simulink model "foot"  (R2014b)
settings: Solver=ode45  StartTime=0.0  StopTime=1  RelTol=1e-3
undefined symbols (not defined in the file or in its folder): MX28_inertia, MX28_Te, X, Y, Z
libraries: sm_lib x10, nesl_utility x7
settings Model: Creator=florent  LastModifiedBy=florent
settings DebuggingCC: IntegerOverflowMsg=none  ParameterDowncastMsg=warning  ParameterPrecisionLossMsg=none  ParameterTunabilityLossMsg=none  StateNameClashWarn=warning  IntegerSaturationMsg=none

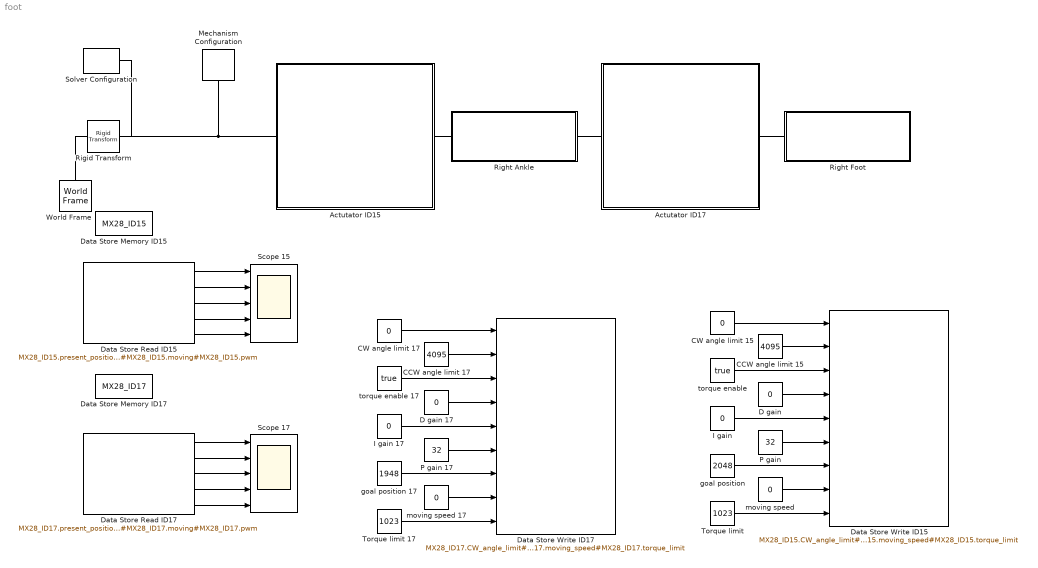
== system foot ==
  Actutator ID15 : Subsystem
  Actutator ID17 : Subsystem
  CCW angle limit 15 : Constant  Value=4095  OutDataTypeStr=int16
  CCW angle limit 17 : Constant  Value=4095  OutDataTypeStr=int16
  CW angle limit 15 : Constant  Value=0  OutDataTypeStr=int16
  CW angle limit 17 : Constant  Value=0  OutDataTypeStr=int16
  D gain : Constant  Value=0  OutDataTypeStr=uint8
  D gain 17 : Constant  Value=0  OutDataTypeStr=uint8
  Data Store Memory ID15 : DataStoreMemory  DataStoreName=MX28_ID15  WriteAfterWriteMsg=error  InitialValue=MX28_default  VectorParams1D=off  OutDataTypeStr=Bus: MX28_bus
  Data Store Memory ID17 : DataStoreMemory  DataStoreName=MX28_ID17  WriteAfterWriteMsg=error  InitialValue=MX28_default  VectorParams1D=off  OutDataTypeStr=Bus: MX28_bus
  Data Store Read ID15 : DataStoreRead  DataStoreName=MX28_ID15  SampleTime=0.001  DataStoreElements=MX28_ID15.present_position#MX28_ID15.present_speed#MX28_ID15.present_load#MX28_ID15.moving#MX28_ID15.pwm
  Data Store Read ID17 : DataStoreRead  DataStoreName=MX28_ID17  SampleTime=0.001  DataStoreElements=MX28_ID17.present_position#MX28_ID17.present_speed#MX28_ID17.present_load#MX28_ID17.moving#MX28_ID17.pwm
  Data Store Write ID15 : DataStoreWrite  DataStoreName=MX28_ID15  DataStoreElements=MX28_ID15.CW_angle_limit#MX28_ID15.CCW_angle_limit#MX28_ID15.torque_enable#MX28_ID15.D_gain#MX28_ID15.I_gain#MX28_ID15.P_gain#MX28_ID15.goal_position#MX28_ID15.moving_speed#MX28_ID15.torque_limit
  Data Store Write ID17 : DataStoreWrite  DataStoreName=MX28_ID17  DataStoreElements=MX28_ID17.CW_angle_limit#MX28_ID17.CCW_angle_limit#MX28_ID17.torque_enable#MX28_ID17.D_gain#MX28_ID17.I_gain#MX28_ID17.P_gain#MX28_ID17.goal_position#MX28_ID17.moving_speed#MX28_ID17.torque_limit
  I gain : Constant  Value=0  OutDataTypeStr=uint8
  I gain 17 : Constant  Value=0  OutDataTypeStr=uint8
  Mechanism Configuration : sm_lib/Utilities/Mechanism Configuration  UniformGravity=Constant  GravityVector=[0 -9.80665 0]  GravityUnits=m/s^2  LinearizationDelta=0.001  BlockFunction=simmechanics.library.utilities.mechanism_configuration
  P gain : Constant  Value=32  OutDataTypeStr=uint8
  P gain 17 : Constant  Value=32  OutDataTypeStr=uint8
  Right Ankle : Subsystem
      mask init:
      | [ModelDir,~,~] = fileparts(which(gcs));
      | 
      | Block = [gcb '/Solid'];
      | STLFileName = [ModelDir filesep 'STL' filesep 'Right_Ankle.STL'];
      | if ~strcmp(get_param(Block,'ExtGeomFileName'),STLFileName)
      |     set_param(Block,'ExtGeomFileName',STLFileName);
      | end
  Right Foot : Subsystem
      mask init:
      | [ModelDir,~,~] = fileparts(which(gcs));
      | 
      | Block = [gcb '/Solid'];
      | STLFileName = [ModelDir filesep 'STL' filesep 'Right_Foot.STL'];
      | if ~strcmp(get_param(Block,'ExtGeomFileName'),STLFileName)
      |     set_param(Block,'ExtGeomFileName',STLFileName);
      | end
  Rigid Transform : sm_lib/Frames and Transforms/Rigid Transform  TranslationMethod=Cartesian  TranslationLengthUnit=m  TranslationStandardAxis=+Z  TranslationStandardOffset=0  TranslationCartesianOffset=[0 -0.001 0]  TranslationROffset=0  TranslationROffsetUnits=m  TranslationZOffset=0  TranslationZOffsetUnits=m  TranslationThetaOffset=0  TranslationThetaOffsetUnits=deg  RotationMethod=AlignedAxes  RotationAngleUnits=deg  RotationStandardAxis=+Z  RotationAngle=0  RotationArbitraryAxis=[0 0 1]  FollAlignAxisA=+Z  BaseAlignAxisA=+X  FollAlignAxisB=+Y  BaseAlignAxisB=+Z  RotationMatrix=[1 0 0; 0 1 0; 0 0 1]  BlockFunction=simmechanics.library.frames_transforms.rigid_transform
  Scope 15 : Scope  NumInputPorts=5
      settings: YMin=-5~0~-5~-5~-5  YMax=5~650~5~5~5
  Scope 17 : Scope  NumInputPorts=5
      settings: YMin=-5~0~-5~-5~-5  YMax=5~650~5~5~5
  Solver Configuration : nesl_utility/Solver Configuration  PhysicalDomain=network_engine_domain  SubClassName=solver  LeftPortType=input  RightPortType=generic  Accelerate=off  Tones=[]  Harmonics=[]  SimulateNoise=off  Profile=off  UseLocalSampling=off  EnableSwitchedLinearOptims=on  FrequencyDomain=off  UseCCode=off  RelTol=0.001  AbsTol=1e-06  MinStep=1e-09  ToWorkspace=off  DoDC=off  ResidualTolerance=1e-09  UseLocalSolver=off  LocalSolverChoice=NE_BACKWARD_EULER_ADVANCER  LocalSolverSampleTime=0.001  DoFixedCost=off  MaxNonlinIter=3  MaxModeIter=2  LinearAlgebra=Sparse  DelaysMemoryBudget=1024  AutomaticFiltering=on  FilteringTimeConstant=0.001
  Torque limit : Constant  Value=1023  OutDataTypeStr=int16
  Torque limit 17 : Constant  Value=1023  OutDataTypeStr=int16
  World Frame : sm_lib/Frames and Transforms/World Frame  BlockFunction=simmechanics.library.frames_transforms.world_frame
  goal position : Constant  Value=2048  OutDataTypeStr=int16
  goal position 17 : Constant  Value=1948  OutDataTypeStr=int16
  moving speed : Constant  Value=0  OutDataTypeStr=int16
  moving speed 17 : Constant  Value=0  OutDataTypeStr=int16
  torque enable : Constant  Value=true  OutDataTypeStr=boolean
  torque enable 17 : Constant  Value=true  OutDataTypeStr=boolean
  wires:
  Data Store Read ID15/1 -> Scope 15/1
  Data Store Read ID15/2 -> Scope 15/2
  Data Store Read ID15/3 -> Scope 15/3
  Data Store Read ID15/4 -> Scope 15/4
  Data Store Read ID15/5 -> Scope 15/5
  Data Store Read ID17/1 -> Scope 17/1
  Data Store Read ID17/2 -> Scope 17/2
  Data Store Read ID17/3 -> Scope 17/3
  Data Store Read ID17/4 -> Scope 17/4
  Data Store Read ID17/5 -> Scope 17/5
  Torque limit 17/1 -> Data Store Write ID17/9
  moving speed 17/1 -> Data Store Write ID17/8
  goal position 17/1 -> Data Store Write ID17/7
  P gain 17/1 -> Data Store Write ID17/6
  I gain 17/1 -> Data Store Write ID17/5
  D gain 17/1 -> Data Store Write ID17/4
  torque enable 17/1 -> Data Store Write ID17/3
  CW angle limit 17/1 -> Data Store Write ID17/1
  CCW angle limit 17/1 -> Data Store Write ID17/2
  Torque limit/1 -> Data Store Write ID15/9
  moving speed/1 -> Data Store Write ID15/8
  goal position/1 -> Data Store Write ID15/7
  P gain/1 -> Data Store Write ID15/6
  I gain/1 -> Data Store Write ID15/5
  D gain/1 -> Data Store Write ID15/4
  torque enable/1 -> Data Store Write ID15/3
  CCW angle limit 15/1 -> Data Store Write ID15/2
  CW angle limit 15/1 -> Data Store Write ID15/1
  connections:
  Mechanism Configuration/RConn1 -- Rigid Transform/RConn1 -- Solver Configuration/RConn1 -- Actutator ID15/LConn1
  Actutator ID15/RConn1 -- Right Ankle/LConn1
  Actutator ID17/LConn1 -- Right Ankle/RConn1
  Actutator ID17/RConn1 -- Right Foot/LConn1
  Rigid Transform/LConn1 -- World Frame/RConn1

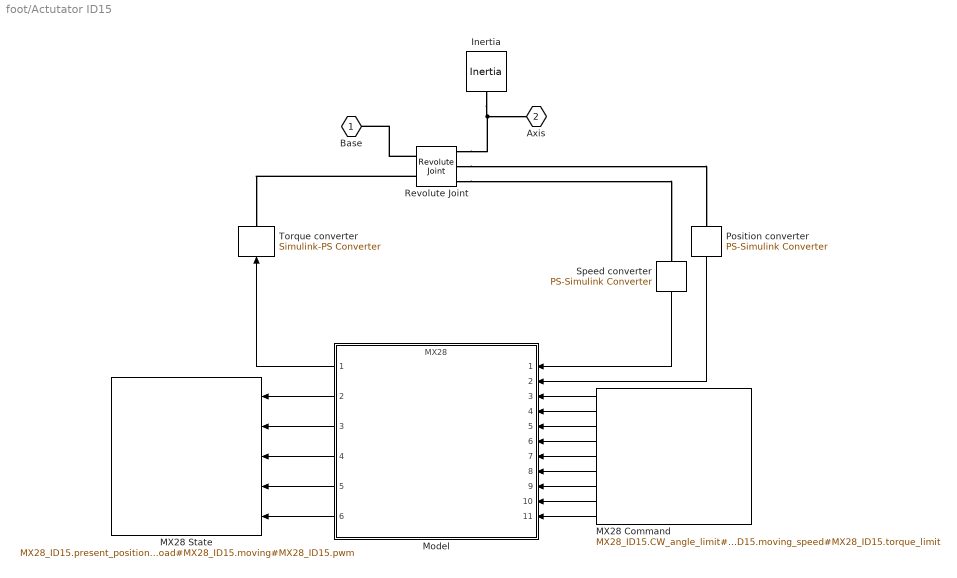
== system foot/Actutator ID15 ==
  Inertia : sm_lib/Body Elements/Inertia  InertiaType=Custom  Mass=1  MassUnits=g  CenterOfMass=[0 0 0]  CenterOfMassUnits=m  MomentsOfInertia=[0 0 MX28_inertia]  MomentsOfInertiaUnits=kg*m^2  ProductsOfInertia=[0 0 0]  ProductsOfInertiaUnits=kg*m^2  BlockFunction=simmechanics.library.body_elements.inertia
  MX28 Command : DataStoreRead  DataStoreName=MX28_ID15  SampleTime=MX28_Te  DataStoreElements=MX28_ID15.CW_angle_limit#MX28_ID15.CCW_angle_limit#MX28_ID15.torque_enable#MX28_ID15.D_gain#MX28_ID15.I_gain#MX28_ID15.P_gain#MX28_ID15.goal_position#MX28_ID15.moving_speed#MX28_ID15.torque_limit
  MX28 State : DataStoreWrite  DataStoreName=MX28_ID15  DataStoreElements=MX28_ID15.present_position#MX28_ID15.present_speed#MX28_ID15.present_load#MX28_ID15.moving#MX28_ID15.pwm
  Model : ModelReference  ModelNameDialog=MX28.slx  SimulationMode=Normal  ModelReferenceVersion=1.66  CopyOfModelName=MX28.slx  DefaultDataLogging=on
  Position converter : nesl_utility/PS-Simulink Converter  PhysicalDomain=network_engine_domain  SubClassName=ps_output  LeftPortType=input  RightPortType=output  PseudoPeriodic=off  Frequencies=[]  Unit=rad  AffineConversion=off
  Revolute Joint : sm_lib/Joints/Revolute Joint  SenseConstraintForce=off  SenseConstraintForceX=off  SenseConstraintForceY=off  SenseConstraintForceZ=off  SenseConstraintTorque=off  SenseConstraintTorqueX=off  SenseConstraintTorqueY=off  SenseConstraintTorqueZ=off  SenseTotalForce=off  SenseTotalForceX=off  SenseTotalForceY=off  SenseTotalForceZ=off  SenseTotalTorque=off  SenseTotalTorqueX=off  SenseTotalTorqueY=off  SenseTotalTorqueZ=off  CompositeWrenchDir=FollowerOnBase  CompositeWrenchFrame=BaseFrame  EquilibriumPosition=0  EquilibriumPositionUnits=deg  SpringStiffness=0  SpringStiffnessUnits=N*m/deg  DampingCoefficient=MX28_lub_friction  DampingCoefficientUnits=N*m/(rad/s)  TorqueActuationMode=InputTorque  MotionActuationMode=ComputedMotion  SensePosition=on  SenseVelocity=on  SenseAcceleration=off  SenseTorqueForce=off  PositionTargetValue=MX28_init_position  PositionTargetValueUnits=rad  PositionTargetSpecify=on  PositionTargetPriority=High  VelocityTargetValue=MX28_init_speed  VelocityTargetValueUnits=rad/s  VelocityTargetSpecify=on  VelocityTargetPriority=High  BlockFunction=simmechanics.library.joints.revolute_joint
  Speed converter : nesl_utility/PS-Simulink Converter  PhysicalDomain=network_engine_domain  SubClassName=ps_output  LeftPortType=input  RightPortType=output  PseudoPeriodic=off  Frequencies=[]  Unit=rad/s  AffineConversion=off
  Torque converter : nesl_utility/Simulink-PS Converter  PhysicalDomain=network_engine_domain  SubClassName=ps_input  LeftPortType=input  RightPortType=output  PseudoPeriodic=off  Frequencies=[]  NoiseDistribution=none  NoiseParameters=[]  Unit=N*m  AffineConversion=off  InputFiltering=off  SimscapeFilterOrder=1  InputFilterTimeConstant=0.001  UdotUserProvided=1
  Base : PMIOPort  Port=1  Side=Left
  Axis : PMIOPort  Port=2  Side=Right
  wires:
  Model/4 -> MX28 State/3
  Model/2 -> MX28 State/1
  Model/5 -> MX28 State/4
  Model/3 -> MX28 State/2
  Model/1 -> Torque converter/1
  Speed converter/1 -> Model/1
  Position converter/1 -> Model/2
  MX28 Command/3 -> Model/5
  MX28 Command/6 -> Model/8
  MX28 Command/4 -> Model/6
  MX28 Command/5 -> Model/7
  MX28 Command/7 -> Model/9
  MX28 Command/2 -> Model/4
  MX28 Command/1 -> Model/3
  Model/6 -> MX28 State/5
  MX28 Command/8 -> Model/10
  MX28 Command/9 -> Model/11
  connections:
  Inertia/RConn1 -- Axis/RConn1 -- Revolute Joint/RConn1
  Revolute Joint/RConn2 -- Position converter/LConn1
  Revolute Joint/LConn2 -- Torque converter/RConn1
  Revolute Joint/RConn3 -- Speed converter/LConn1
  Revolute Joint/LConn1 -- Base/RConn1

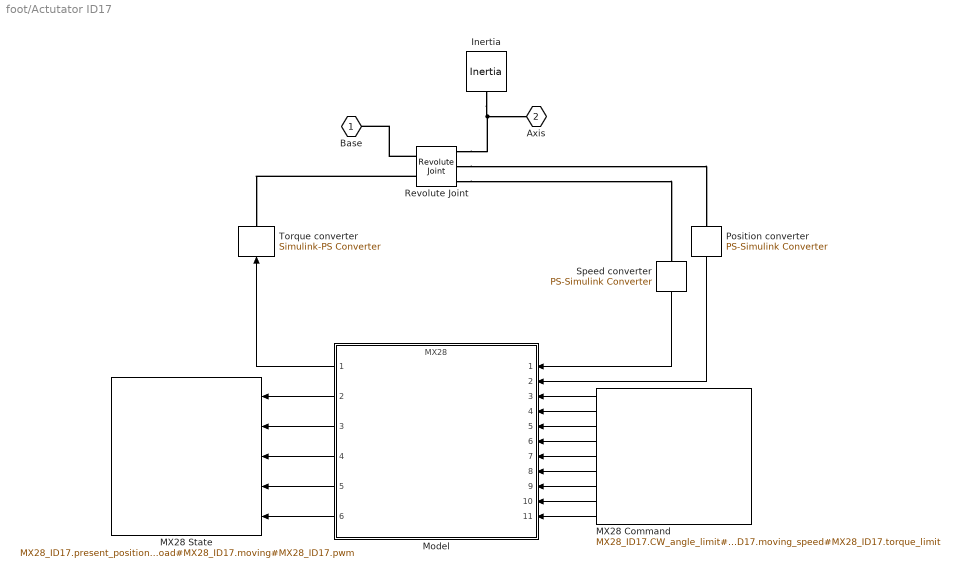
== system foot/Actutator ID17 ==
  Inertia : sm_lib/Body Elements/Inertia  InertiaType=Custom  Mass=1  MassUnits=g  CenterOfMass=[0 0 0]  CenterOfMassUnits=m  MomentsOfInertia=[0 0 MX28_inertia]  MomentsOfInertiaUnits=kg*m^2  ProductsOfInertia=[0 0 0]  ProductsOfInertiaUnits=kg*m^2  BlockFunction=simmechanics.library.body_elements.inertia
  MX28 Command : DataStoreRead  DataStoreName=MX28_ID17  SampleTime=MX28_Te  DataStoreElements=MX28_ID17.CW_angle_limit#MX28_ID17.CCW_angle_limit#MX28_ID17.torque_enable#MX28_ID17.D_gain#MX28_ID17.I_gain#MX28_ID17.P_gain#MX28_ID17.goal_position#MX28_ID17.moving_speed#MX28_ID17.torque_limit
  MX28 State : DataStoreWrite  DataStoreName=MX28_ID17  DataStoreElements=MX28_ID17.present_position#MX28_ID17.present_speed#MX28_ID17.present_load#MX28_ID17.moving#MX28_ID17.pwm
  Model : ModelReference  ModelNameDialog=MX28.slx  SimulationMode=Normal  ModelReferenceVersion=1.66  CopyOfModelName=MX28.slx  DefaultDataLogging=on
  Position converter : nesl_utility/PS-Simulink Converter  PhysicalDomain=network_engine_domain  SubClassName=ps_output  LeftPortType=input  RightPortType=output  PseudoPeriodic=off  Frequencies=[]  Unit=rad  AffineConversion=off
  Revolute Joint : sm_lib/Joints/Revolute Joint  SenseConstraintForce=off  SenseConstraintForceX=off  SenseConstraintForceY=off  SenseConstraintForceZ=off  SenseConstraintTorque=off  SenseConstraintTorqueX=off  SenseConstraintTorqueY=off  SenseConstraintTorqueZ=off  SenseTotalForce=off  SenseTotalForceX=off  SenseTotalForceY=off  SenseTotalForceZ=off  SenseTotalTorque=off  SenseTotalTorqueX=off  SenseTotalTorqueY=off  SenseTotalTorqueZ=off  CompositeWrenchDir=FollowerOnBase  CompositeWrenchFrame=BaseFrame  EquilibriumPosition=0  EquilibriumPositionUnits=deg  SpringStiffness=0  SpringStiffnessUnits=N*m/deg  DampingCoefficient=MX28_lub_friction  DampingCoefficientUnits=N*m/(rad/s)  TorqueActuationMode=InputTorque  MotionActuationMode=ComputedMotion  SensePosition=on  SenseVelocity=on  SenseAcceleration=off  SenseTorqueForce=off  PositionTargetValue=MX28_init_position  PositionTargetValueUnits=rad  PositionTargetSpecify=on  PositionTargetPriority=High  VelocityTargetValue=MX28_init_speed  VelocityTargetValueUnits=rad/s  VelocityTargetSpecify=on  VelocityTargetPriority=High  BlockFunction=simmechanics.library.joints.revolute_joint
  Speed converter : nesl_utility/PS-Simulink Converter  PhysicalDomain=network_engine_domain  SubClassName=ps_output  LeftPortType=input  RightPortType=output  PseudoPeriodic=off  Frequencies=[]  Unit=rad/s  AffineConversion=off
  Torque converter : nesl_utility/Simulink-PS Converter  PhysicalDomain=network_engine_domain  SubClassName=ps_input  LeftPortType=input  RightPortType=output  PseudoPeriodic=off  Frequencies=[]  NoiseDistribution=none  NoiseParameters=[]  Unit=N*m  AffineConversion=off  InputFiltering=off  SimscapeFilterOrder=1  InputFilterTimeConstant=0.001  UdotUserProvided=1
  Base : PMIOPort  Port=1  Side=Left
  Axis : PMIOPort  Port=2  Side=Right
  wires:
  Model/4 -> MX28 State/3
  Model/2 -> MX28 State/1
  Model/5 -> MX28 State/4
  Model/3 -> MX28 State/2
  Model/1 -> Torque converter/1
  Speed converter/1 -> Model/1
  Position converter/1 -> Model/2
  MX28 Command/3 -> Model/5
  MX28 Command/6 -> Model/8
  MX28 Command/4 -> Model/6
  MX28 Command/5 -> Model/7
  MX28 Command/7 -> Model/9
  MX28 Command/2 -> Model/4
  MX28 Command/1 -> Model/3
  Model/6 -> MX28 State/5
  MX28 Command/8 -> Model/10
  MX28 Command/9 -> Model/11
  connections:
  Inertia/RConn1 -- Axis/RConn1 -- Revolute Joint/RConn1
  Revolute Joint/RConn3 -- Speed converter/LConn1
  Revolute Joint/LConn2 -- Torque converter/RConn1
  Revolute Joint/RConn2 -- Position converter/LConn1
  Revolute Joint/LConn1 -- Base/RConn1

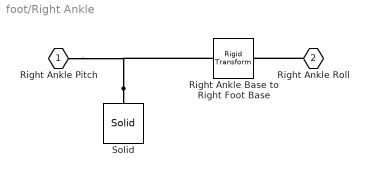
== system foot/Right Ankle ==
  Right Ankle Base to Right Foot Base : sm_lib/Frames and Transforms/Rigid Transform  TranslationMethod=Cartesian  TranslationLengthUnit=mm  TranslationStandardAxis=+Z  TranslationStandardOffset=0  TranslationCartesianOffset=[-19.35 0 -24]  TranslationROffset=0  TranslationROffsetUnits=m  TranslationZOffset=0  TranslationZOffsetUnits=m  TranslationThetaOffset=0  TranslationThetaOffsetUnits=deg  RotationMethod=AlignedAxes  RotationAngleUnits=deg  RotationStandardAxis=+Z  RotationAngle=0  RotationArbitraryAxis=[0 0 1]  FollAlignAxisA=+X  BaseAlignAxisA=+Z  FollAlignAxisB=+Y  BaseAlignAxisB=-Y  RotationMatrix=[1 0 0; 0 1 0; 0 0 1]  BlockFunction=simmechanics.library.frames_transforms.rigid_transform
  Solid : sm_lib/Body Elements/Solid  InertiaType=Custom  Mass=166.79  MassUnits=g  CenterOfMass=[-18.06 -11.21 -24.20]  CenterOfMassUnits=mm  MomentsOfInertia=[6948 12212 11817]  MomentsOfInertiaUnits=g*mm^2  ProductsOfInertia=[-194 117 4006]  ProductsOfInertiaUnits=g*mm^2  DensityBased=on  Density=1000  DensityUnits=kg/(m^3)  GraphicType=FromGeometry  MarkerShape=Sphere  MarkerSize=10  MarkerSizeUnits=m  GraphicVisPropType=SimpleVisualProperties  GraphicDiffuseColor=[0.5 0.5 0.5]  GraphicSpecularColor=[0.5 0.5 0.5 1.0]  GraphicAmbientColor=[0.15 0.15 0.15 1.0]  GraphicEmissiveColor=[0.0 0.0 0.0 1.0]  GraphicShininess=75  GraphicOpacity=1.0  GeometryShape=FromFile  RectangleSize=[1 1]  RectangleSizeUnits=m  BrickDimensions=[1 1 1]  BrickDimensionUnits=m  CylinderRadius=1  CylinderRadiusUnits=m  CylinderLength=1  CylinderLengthUnits=m  SphereRadius=1  SphereRadiusUnits=m  EllipsoidRadii=[1 1 1]  EllipsoidRadiiUnits=m  ExtrusionCrossSection=[1 1; -1 1; -1 -1; 1 -1]  ExtrusionCrossSectionUnits=m  ExtrusionLength=1  ExtrusionLengthUnits=m  PolygonNumSides=3  PolygonOuterRadius=1  PolygonOuterRadiusUnits=m  ExtGeomFileType=STL  ExtGeomFileName=D:\Ker Lann\systemes\darwin\kinematics\STL\Right_Ankle.STL  ExtGeomFileUnits=mm  RevolutionCrossSection=[1 1; 1 -1; 2 -1; 2 1]  RevolutionCrossSectionUnits=m  RevolutionExtent=Full  RevolutionAngle=180  RevolutionAngleUnits=deg  BlockFunction=simmechanics.library.body_elements.solid
  Right Ankle Pitch : PMIOPort  Port=1  Side=Left
  Right Ankle Roll : PMIOPort  Port=2  Side=Right
  connections:
  Solid/RConn1 -- Right Ankle Base to Right Foot Base/LConn1 -- Right Ankle Pitch/RConn1
  Right Ankle Roll/RConn1 -- Right Ankle Base to Right Foot Base/RConn1

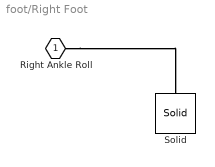
== system foot/Right Foot ==
  Solid : sm_lib/Body Elements/Solid  InertiaType=Custom  Mass=76.78  MassUnits=g  CenterOfMass=[7.76 24.5 17.25]  CenterOfMassUnits=mm  MomentsOfInertia=[69069 85303 36676]  MomentsOfInertiaUnits=g*mm^2  ProductsOfInertia=[4062 778 2754]  ProductsOfInertiaUnits=g*mm^2  DensityBased=on  Density=1000  DensityUnits=kg/(m^3)  GraphicType=FromGeometry  MarkerShape=Sphere  MarkerSize=10  MarkerSizeUnits=m  GraphicVisPropType=SimpleVisualProperties  GraphicDiffuseColor=[0.5 0.5 0.5]  GraphicSpecularColor=[0.5 0.5 0.5 1.0]  GraphicAmbientColor=[0.15 0.15 0.15 1.0]  GraphicEmissiveColor=[0.0 0.0 0.0 1.0]  GraphicShininess=75  GraphicOpacity=1.0  GeometryShape=FromFile  RectangleSize=[1 1]  RectangleSizeUnits=m  BrickDimensions=[1 1 1]  BrickDimensionUnits=m  CylinderRadius=1  CylinderRadiusUnits=m  CylinderLength=1  CylinderLengthUnits=m  SphereRadius=1  SphereRadiusUnits=m  EllipsoidRadii=[1 1 1]  EllipsoidRadiiUnits=m  ExtrusionCrossSection=[1 1; -1 1; -1 -1; 1 -1]  ExtrusionCrossSectionUnits=m  ExtrusionLength=1  ExtrusionLengthUnits=m  PolygonNumSides=3  PolygonOuterRadius=1  PolygonOuterRadiusUnits=m  ExtGeomFileType=STL  ExtGeomFileName=D:\Ker Lann\systemes\darwin\kinematics\STL\Right_Foot.STL  ExtGeomFileUnits=mm  RevolutionCrossSection=[1 1; 1 -1; 2 -1; 2 1]  RevolutionCrossSectionUnits=m  RevolutionExtent=Full  RevolutionAngle=180  RevolutionAngleUnits=deg  BlockFunction=simmechanics.library.body_elements.solid
  Right Ankle Roll : PMIOPort  Port=1  Side=Left
  connections:
  Right Ankle Roll/RConn1 -- Solid/RConn1
